simulink model "s_f_withnoise"  (R2018b)
settings: Solver=VariableStepAuto  StartTime=0.0  StopTime=30.0  RelTol=1e-3
values from neighbouring files (symbols this model uses):
  A = [0,1,0,0 ; 0,-0.1818,2.6727,0; 0,0,0,1;0,-0.4545,31.1818,0;]    [rlocus.m]
  B = [0;1.8182;0;4.5455]    [rlocus.m]
  C = [0,0,1,0]    [rlocus.m]
  D = 0    [rlocus.m]
  K = place(A,B,p)    [rlocus.m]
libraries: simulink x2
settings Model: Creator=Tara  LastModifiedBy=Tara

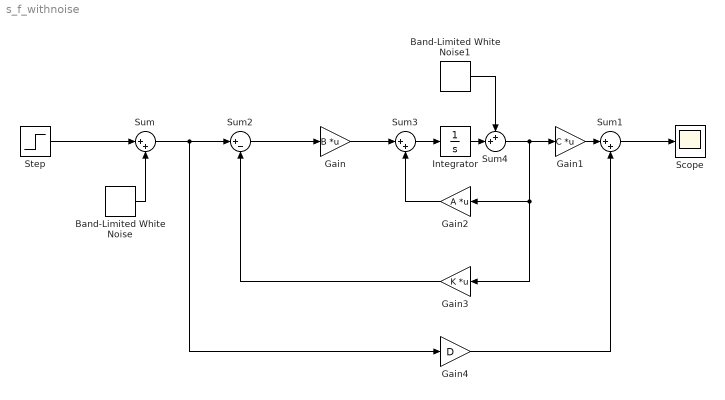
== system s_f_withnoise ==
  Band-Limited White Noise : simulink/Sources/Band-Limited White Noise  Cov=[0.000001]  Ts=0.1  seed=[23341]
  Band-Limited White Noise1 : simulink/Sources/Band-Limited White Noise  Cov=[0.00000001]  Ts=0.1  seed=[23341]
  Gain : Gain  Gain=B  Multiplication=Matrix(K*u)
  Gain1 : Gain  Gain=C  Multiplication=Matrix(K*u)
  Gain2 : Gain  Gain=A  Multiplication=Matrix(K*u)
  Gain3 : Gain  Gain=K  Multiplication=Matrix(K*u)
  Gain4 : Gain  Gain=D
  Integrator : Integrator
  Scope : Scope
  Step : Step  SampleTime=0
  Sum : Sum  Inputs=|++
  Sum1 : Sum  Inputs=|++
  Sum2 : Sum  Inputs=|+-
  Sum3 : Sum  Inputs=|++
  Sum4 : Sum  Inputs=++|
  wires:
  Gain/1 -> Sum3/1
  Sum2/1 -> Gain/1
  Sum3/1 -> Integrator/1
  Gain1/1 -> Sum1/1
  Sum1/1 -> Scope/1
  Gain2/1 -> Sum3/2
  Gain3/1 -> Sum2/2
  Gain4/1 -> Sum1/2
  Step/1 -> Sum/1
  Band-Limited White Noise/1 -> Sum/2
  Sum/1 -> Gain4/1, Sum2/1
  Sum4/1 -> Gain3/1, Gain2/1, Gain1/1
  Band-Limited White Noise1/1 -> Sum4/1
  Integrator/1 -> Sum4/2
